simulink model "hexa_tilted_EHGO_ASMC"  (R2023a)
settings: Solver=ode1  StartTime=0.0  StopTime=tf  FixedStep=0.01  RelTol=1e-3
model workspace (MAT data in the model file):
  hover_2m = [0  0  0  0  0  0; 0  0  0  0  0  0; 2  2  2  2  2  2; 0  0  0  0  0  0; 0  0  0  0  0  0; 0  0  0  0  0  0]
  tf = Simulink.Parameter
  tf.Value = 60
  tf.DataType = 'auto'
  tf.Complexity = 'real'
  tf.Dimensions = [1 1]
  tray0 = [0  0  0  0  0  0; 0  0  0  0  0  0; 0  5  5  5  5  0; 0  0  0  0  0  0; 0  0  0  0  0  0; 0  0  0  0  0  0]
  tray1 = [0  0  0  0  0  0; 0  0  0  0  0  0; 0  5  2.5  5  2.5  0; 0  0  0  0  0  0; 0  0  0  0  0  0; 0  0  0  0  0  0]
  tray2 = [0  2  2  -2  -2  0; 0  0  -2  -2  2  0; 0  5  2.5  5  2.5  0; 0  0  0  0  0  0; 0  0  0  0  0  0; 0  0  0  0  0  0]
  tray3 = [0  2  2  -2  -2  0; 0  0  -2  -2  2  0; 0  5  2.5  5  2.5  0; 0  0  0  0  0  0; 0  0  0  0  0  0; 0  0  0.785  1.57  0.785  0]
  tray4 = [0  2  2  -2  -2  0; 0  0  -2  -2  2  0; 0  5  2.5  5  2.5  0; 0  0.15  0.15  0.15  0.15  0; 0  0  0  0  0  0; 0  0  0.785  1.57  0.785  0]
  tray5 = [0  0  0  0  0  0; 0  0  0  0  0  0; 0  5  2.5  5  2.5  0; 0  0.15  0.15  0  0  0; 0  0  0.15  0.15  0  0; 0  0  0  0  0  0]
  tray_yaw = [0  0  0  0  0  0; 0  0  0  0  0  0; 0  5  2.5  5  2.5  0; 0  0  0  0  0  0; 0  0  0  0  0  0; 0  0  0.785  1.57  0.785  0]
undefined symbols (not defined in the file or in its folder): F, Light, MIL
libraries: matrix_library x1, aerolibutil x1, simulink x1, robotcorelib x1, sharedtransform x1, aerolibwind2 x1, SignalEditorBlockLib x1
settings Model: Creator=adan  LastModifiedBy=Adan Daniel
settings OptimizationCC: ReuseModelBlockBuffer=off

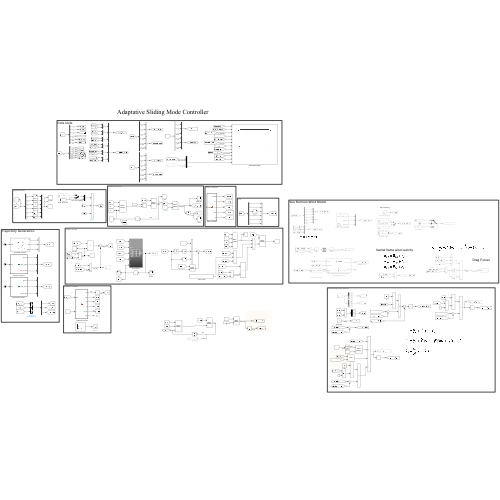
[thumbnail: Simulink's stored preview of the top-level diagram]
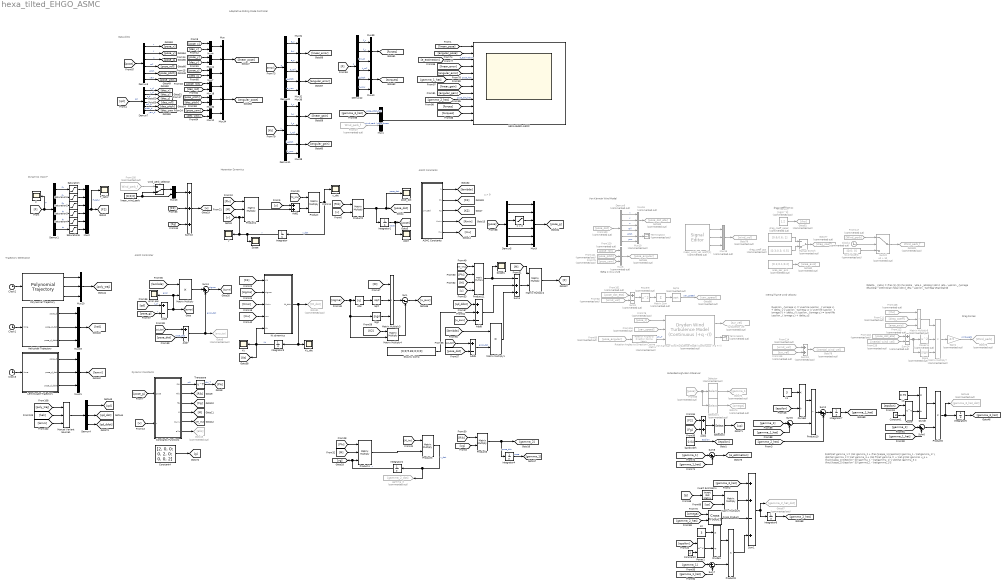
== system hexa_tilted_EHGO_ASMC ==
  note: $\dot\hat \gamma_1 = \hat \gamma_2 + \frac{\kappa_1}{\epsilon}(\gamma_1 - \hat\gamma_1) \\ \dot\hat \gamma_2 = \hat \gamma_3 + \hat f(\hat \gamma, t) + \hat g(\hat \gamma) u_p + \frac{\kappa_2}{\epsilon^2}(\gamma_1 - \hat\gamma_1) \\ \dot\hat \gamma_3 = \frac{\kappa_3}{\epsilon^3}(\gamma_1 - \hat\gamma_1)$
  note: z > 0
  note: Adaptative Sliding Mode Controller
  note: ASMC Constants
  note: ASMC Controller
  note: Dynamic Constants
  note: Hexarotor Dynamics
  note: Dynamics Input F
  note: Data plots
  note: Trajectory Generation
  note: drag coeff from []
  note: $\upsilon _{\omega x} = \overline \upsilon _{ \omega x} + \delta_u \\ \upsilon _{\omega y} = \overline \upsilon _{ \omega y} + \delta_u \\ \upsilon _{\omega z} = \overline \upsilon _{ \omega z} + \delta_u$
  note: $\eta = \{x,y,z\}$
  note: Inertial frame wind velocity
  note: $\Delta _ {\eta} = \frac{1}{2}\rho \alpha _ \eta A _\eta\big (\dot d_\eta - \upsilon _{\omega \eta}\big)^2\text{sign }\big (\dot d_\eta - \upsilon _{\omega \eta}\big)$$
  note: Von Kármán Wind Model
  note: Drag Forces
  note: Extended High-Gain Observer
  ASMC Constants : MATLAB Function  TreatAsAtomicUnit=on
  Abs : Abs  SaturateOnIntegerOverflow=off
  Add1 : Sum
  Add2 : Sum
  Add6 : Sum  Inputs=+-
  Add7 : Sum  Inputs=+-
  Add8 : Sum  Inputs=++-
  Add9 : Sum  Inputs=+-
  Clock1 : Clock
  Clock2 : Clock
  Clock3 : Clock
  Clock4 : Clock  Commented=on
  Constant1 : Constant  Value=3
  Constant2 : Constant  Value=2
  Constant4 : Constant  Value=[2, 0, 0; 0, 2, 0; 0, 0, 2]
  Constants Functions : MATLAB Function  TreatAsAtomicUnit=on
  Cross Product : matrix_library/Cross Product
  Demux{1,3,5,7..8,11..12} (7 alike) : Demux  Outputs=6
  Demux4 : Demux  Outputs=3
  Demux6 : Demux  Commented=on  Outputs=6
  Divide : Product  Inputs=*/
  Divide1 : Product  Inputs=*/
  Divide2 : Product  Inputs=*/
  F : Scope
  F_satur : Scope
  From100 : From  Commented=on  GotoTag=pose_dot
  From101 : From  Commented=on  GotoTag=pose_dot_eta
  From104 : From  Commented=on  GotoTag=uav_speed
  From105 : From  Commented=on  GotoTag=Wind_perb_f  TagVisibility=global
  From106 : From  Commented=on  GotoTag=rho
  From111 : From  Commented=on  GotoTag=drag_coeff
  From112 : From  Commented=on  GotoTag=area_axis
  From114 : From  Commented=on  GotoTag=wind_vel
  From115 : From  Commented=on  GotoTag=tur_vel
  From117 : From  Commented=on  GotoTag=Wind_perb
  From118 : From  Commented=on  GotoTag=pose_dot_eta
  From120 : From  Commented=on  GotoTag=pose_roll
  From121 : From  Commented=on  GotoTag=pose_pitch
  From126 : From  Commented=on  GotoTag=inertial_wind_vel
  From27 : From  Commented=on  GotoTag=Wind_perb_f  TagVisibility=global
  From65 : From  Commented=on  GotoTag=pose
  From75 : From  Commented=on  GotoTag=pose_yaw
  From76 : From  Commented=on  GotoTag=pose_z
  From82 : From  Commented=on  GotoTag=wind_vel
  From83 : From  Commented=on  GotoTag=pose_angular
  Gain1 : Gain  Commented=on  Gain=-0.5
  Goto15 : Goto  Commented=on  GotoTag=allo
  Goto31 : Goto  Commented=on  GotoTag=Kt_dot
  Goto39 : Goto  Commented=on  GotoTag=Wind_perb_f  TagVisibility=global
  Goto45 : Goto  Commented=on  GotoTag=gamma_3_hat_dot
  Goto6 : Goto  Commented=on  GotoTag=error_dot
  Goto67 : Goto  Commented=on  GotoTag=gamma_2_hat_dot
  Goto70 : Goto  Commented=on  GotoTag=gamma_1
  Goto74 : Goto  Commented=on  GotoTag=omega
  Goto76 : Goto  Commented=on  GotoTag=Wind_perb
  Goto77 : Goto  Commented=on  GotoTag=drag_coeff
  Goto78 : Goto  Commented=on  GotoTag=inertial_wind_vel
  Goto79 : Goto  Commented=on  GotoTag=wind_vel
  Goto80 : Goto  Commented=on  GotoTag=uav_speed
  Goto81 : Goto  Commented=on  GotoTag=rho
  Goto82 : Goto  Commented=on  GotoTag=area_axis
  Goto83 : Goto  Commented=on  GotoTag=pose_dot_eta
  Goto84 : Goto  Commented=on  GotoTag=pose_angular
  Gravity Comp : Constant  Value=[0;0;9.81;0;0;0]
  HEXA EHGO-ASMC : Scope  NumInputPorts=12
  Helicoidal Trajectory : MATLAB Function  TreatAsAtomicUnit=on
  Integrator{,1..4} (5 alike) : Integrator  InitialCondition=[0; 0; 0; 0; 0; 0]
  Integrator5 : Integrator  InitialCondition=[0; 0; 0]
  Integrator6 : Integrator  InitialCondition=[0; 0; 0]
  Integrator7 : Integrator  InitialCondition=[0; 0; 0]
  Invert 3x3 Matrix : aerolibutil/Invert  3x3 Matrix
  Kt : Scope
  Kt dynamics : Subsystem
  Kt_dot : Scope
  Lemniscate Trajectory : MATLAB Function  TreatAsAtomicUnit=on
  Manual Variant Source1 : simulink/Signal Routing/Manual Variant Source  NumChoices=3  LabelModeActiveChoice=V_2
  Manual Switch : ManualSwitch  Commented=on  CurrentSetting=0
  Matrix Sum : Sum  Commented=on  Inputs=+
  Matrix Multiply : Product
  Matrix Multiply1 : Product
  Matrix Multiply2 : Product  Multiplication=Matrix(*)
  Matrix Multiply3 : Product  Inputs=3
  Matrix Multiply4 : Product  Multiplication=Matrix(*)
  Matrix Multiply5 : Product  Multiplication=Matrix(*)
  Matrix Multiply6 : Product  Commented=on  Inputs=3
  Matrix Multiply7 : Product  Commented=on  Inputs=3
  Mux{,19..21,31..32,34,36,38..40} (11 alike) : Mux  Inputs=3
  Mux{1,4,7,11..13,18,30} (8 alike) : Mux  Inputs=2
  Mux{5,10,15..16} (4 alike) : Mux  Commented=on  Inputs=3
  Mux2 : Mux  Inputs=6
  Mux9 : Mux  Inputs=6
  Polynomial Trajectory : robotcorelib/Polynomial Trajectory  WaypointSource=Internal  Waypoints=tray1  TimePoints=[ 0, 12, 24, 36, 48, tf ]  TimeInterval=[ 1, 4 ]  Method=Cubic Polynomial  ParameterSource=Internal  VelocityBoundaryCondition=zeros( 6, 6 )  AccelerationBoundaryCondition=zeros( 2, 5 )  SimulateUsing=Interpreted execution
  Power : Math  Operator=pow
  Power1 : Math  Operator=pow
  Power11 : Math  Commented=on  Operator=square
  Power9 : Math  Commented=on  Operator=square
  Product{,2..3,5} (4 alike) : Product  Multiplication=Matrix(*)
  Product1 : Product  Inputs=3  Multiplication=Matrix(*)
  Product10 : Product
  Product11 : Product  Inputs=4  Multiplication=Matrix(*)
  Product4 : Product  Inputs=3  Multiplication=Matrix(*)
  Product6 : Product
  Product8 : Product
  Rotation Angles to Direction Cosine Matrix : sharedtransform/Rotation Angles to Direction Cosine Matrix  Commented=on  rotationOrder=ZYX  aMode=aMode
  Saturation : Saturate  UpperLimit=6  LowerLimit=-6
  Saturation1 : Saturate  UpperLimit=6  LowerLimit=-6
  Saturation2 : Saturate  UpperLimit=5.8*6  LowerLimit=0
  Saturation3 : Saturate
  Saturation4 : Saturate
  Saturation5 : Saturate
  Scope : Scope
  Scope1 : Scope
  Selector : Selector  Commented=on  InputPortWidth=6  IndexOptions=Index vector (dialog)  Indices=[1:3]  OutputSizes=1
  Selector1 : Selector  Commented=on  InputPortWidth=6  IndexOptions=Index vector (dialog)  Indices=[4:6]  OutputSizes=1
  Selector2 : Selector  InputPortWidth=6  IndexOptions=Index vector (dialog)  Indices=[1:3]  OutputSizes=1
  Sign : Signum
  Sign4 : Signum  Commented=on
  Sqrt : Sqrt
  Sqrt4 : Sqrt  Commented=on
  Sum : Sum  Inputs=|--
  Sum1 : Sum  Inputs=++-+
  Sum10 : Sum  Inputs=+++
  Sum13 : Sum  Commented=on
  Sum14 : Sum  Commented=on  Inputs=+-
  Sum2 : Sum  Inputs=|++
  Sum3 : Sum  Inputs=|++
  Sum4 : Sum  Inputs=-++
  Sum{5..8} (4 alike) : Sum  Inputs=|+-
  Sum9 : Sum  Commented=on  Inputs=+-
  Switch : Switch  Commented=on  Criteria=u2 > Threshold  Threshold=10  SaturateOnIntegerOverflow=off  InputSameDT=off
  Terminator1 : Terminator  Commented=on
  Terminator2 : Terminator  Commented=on
  Transpose : Math  Operator=transpose
  Von Karman Wind Turbulence Model (Continuous (+q +r)) : aerolibwind2/Dryden Wind Turbulence Model  (Continuous (+q -r))  Commented=on  units=Metric (MKS)  spec=MIL-F-8785C  model=Continuous Von Karman (+q -r)  W20=15  Wdeg=0  TurbProb=10^-2 - Light  L_high=762  Wingspan=10  ts=0.1  Seed=[23341 23342 23343 23344]  T_on=on
      settings: LibrarySourceBlock=|
      | aerolibwind2/Von Karman Wind Turbulence Model
      | (Continuous (+q +r))
  air density [kg/m^3] : Constant  Commented=on  Value=1.2
  area_per_axis : Constant  Commented=on  Value=[0.1;0.1;0.2]
  bandwidth : Constant  Value=0.04
  drag_coeff_gus : Constant  Commented=on  Value=[0.3;0.3; 0.5]
  drag_coeff_paper : Constant  Commented=on  Value=[0.6;0.6; 1]
  error pos : Scope
  gamma_3 : Goto  Commented=on  GotoTag=gamma_2_dot
  k1 : Constant  Value=3
  k2 : Constant  Value=3
  k3 : Constant  Value=0.75
  linear_wind_perb : Constant  Value=[0;0;0]
  mean_wind_vel_ansft[1] : SignalEditorBlockLib/Signal Editor  Commented=on  FileName=C:\Users\Adan Daniel\Documents\IMT\8Semestre_tec\Diseño e implementación de sistemas mecatronicos\mean_wind_vel_ansft.mat  ActiveScenario=Velocidades_medias_del_viento  ActiveSignal=wean_wind_vel_x  IsBus=off  OutputBusObjectStr=Bus: BusObject  SampleTime=0  Interpolate=off  ZeroCross=off  OutputAfterFinalValue=Setting to zero  Unit=inherit  PreserveSignalName=on  ApplySigPropsToAllScenarios=on
  no wind perb : Constant  Commented=on  Value=[0;0; 0]
  pose : Scope
  pose_dot : Scope
  turbulence_vel : Goto  Commented=on  GotoTag=tur_vel
  v : Scope
  v_dot : Scope
  wind_perb_selector : ManualSwitch  CurrentSetting=0
  z > 0 : Saturate  UpperLimit=100  LowerLimit=0
  wires:
  Saturation/1 -> Mux2/1
  Saturation1/1 -> Mux2/2
  Saturation4/1 -> Mux2/5
  Saturation3/1 -> Mux2/4
  Demux1/6 -> Saturation5/1  "tz"
  Demux1/3 -> Saturation2/1  "Fz"
  [F] -> F/1, Demux1/1  "F"
  Saturation5/1 -> Mux2/6
  Demux1/2 -> Saturation1/1  "Fy"
  Demux1/1 -> Saturation/1  "Fx"
  Demux1/5 -> Saturation4/1  "ty"
  Demux1/4 -> Saturation3/1  "tx"
  Saturation2/1 -> Mux2/3
  Mux2/1 -> [F2], F_satur/1  "F_satur"
  [M] -> Product1/2
  [v] -> Product2/2
  [M_inv] -> Product/1
  Add2/1 -> Product/2
  Product/1 -> v_dot/1, Integrator/1  "v_dot"
  [Rib] -> Product2/1
  Product2/1 -> Integrator1/1, pose_dot/1, [pose_dot]  "pose_dot"
  [Phi] -> Product1/1
  Product1/1 -> Add2/2
  Integrator1/1 -> pose/1, [pose]  "pose"
  Integrator/1 -> Scope/1, v/1, [v], Product1/3  "v"
  [pose_g] -> Constants Functions/1(pose)
  [v] -> Constants Functions/2(v)
  Constants Functions/6(allo) -> Goto15/1
  Constants Functions/3(Fg) -> [Fg]
  Constants Functions/4(M) -> [M]
  Constants Functions/1(Phi) -> Transpose/1  "phi"
  Constants Functions/2(Rib) -> [Rib]
  Transpose/1 -> [Phi]  "phi_T"
  Constants Functions/5(M_inv) -> [M_inv]
  [K1] -> Kt dynamics/1(K1)
  [sigma] -> Kt dynamics/2(sigma)
  [qd] -> Add6/1  "x_d"
  [Kt] -> Matrix Multiply3/1
  [mu] -> Kt dynamics/4(mu)
  Sum3/1 -> [sigma]  "sigma"
  [u_aux] -> Add8/3
  [qd_dot] -> Add9/1
  Add6/1 -> [error], Matrix Multiply/2, error pos/1  "error"
  [lambda] -> Matrix Multiply1/1
  [v] -> Product11/4  "v"
  [M] -> Matrix Multiply2/1
  Matrix Multiply4/1 -> Sum/2
  [pose_dot] -> Add9/2
  Matrix Multiply/1 -> Sum3/1
  [qd_ddot] -> Add8/1
  Add7/1 -> Goto6/1, Sum3/2  "error_dot"
  Matrix Multiply2/1 -> [F]
  [lambda] -> Matrix Multiply/1
  Sum4/1 -> Matrix Multiply2/2
  Product11/1 -> Scope1/1, Sum4/1
  [M] -> Product11/3
  Integrator3/1 -> [Kt], Kt/1, Kt dynamics/5(Kt)  "Kt"
  [pose_dot] -> Add7/2  "pose_dot"
  [K2] -> Matrix Multiply4/1
  Add9/1 -> Matrix Multiply1/2  "error_dot"
  Sign/1 -> Matrix Multiply3/3
  Abs/1 -> Sqrt/1
  [pose_g] -> Add6/2  "x"
  [M_inv] -> Product11/1
  [Kmin] -> Kt dynamics/3(Kmin)
  Add8/1 -> Sum4/2
  Matrix Multiply1/1 -> Sum4/3
  [sigma] -> Matrix Multiply4/2, Sign/1, Abs/1
  Kt dynamics/1(Kt_dot) -> Integrator3/1, Kt_dot/1, Goto31/1
  [Phi] -> Product11/2
  [qd_dot] -> Add7/1
  Matrix Multiply3/1 -> Sum/1
  Sum/1 -> [u_aux]
  ASMC Constants/4(Kmin) -> [Kmin]
  ASMC Constants/3(K2) -> [K2]
  ASMC Constants/5(mu) -> [mu]
  ASMC Constants/2(K1) -> [K1]
  ASMC Constants/1(lambda) -> [lambda]
  Sqrt/1 -> Matrix Multiply3/2
  Demux5/5 -> Mux9/5
  Demux5/6 -> Mux9/6
  Mux9/1 -> [pose_g]
  Demux5/1 -> Mux9/1
  Demux5/3 -> z > 0/1
  Demux5/2 -> Mux9/2
  Demux5/4 -> Mux9/4
  [pose] -> Demux5/1
  z > 0/1 -> Mux9/3
  Gravity Comp/1 -> Add8/2
  k3/1 -> Divide/1
  Power/1 -> Divide/2
  Constant1/1 -> Power/2
  Divide/1 -> Product6/1
  Product6/1 -> Integrator5/1, Goto45/1
  Integrator5/1 -> [gamma_3_hat]
  [des_roll] -> Mux18/2
  Mux11/1 -> Mux/2
  [des_yaw] -> Mux12/2
  [pose_pitch] -> Mux30/1
  [des_z] -> Mux7/2
  Mux4/1 -> Mux/1
  [des_pitch] -> Mux30/2
  Mux7/1 -> Mux/3
  [qd] -> Demux7/1  "qd"
  Demux3/5 -> [pose_pitch]  "pitch"
  Demux3/2 -> [pose_y]  "y"
  Demux8/4 -> Mux32/1  "e_roll"
  Demux8/2 -> Mux31/2  "e_y"
  Demux8/1 -> Mux31/1  "e_x"
  [pose_x] -> Mux4/1
  Demux3/4 -> [pose_roll]  "roll"
  Mux31/1 -> [linear_error]
  Demux7/3 -> [des_z]  "z_d"
  Mux34/1 -> [angular_pose]
  [des_y] -> Mux11/2
  Mux12/1 -> Mux34/3
  Demux3/3 -> [pose_z]  "z"
  [error] -> Demux8/1  "e"
  Demux8/5 -> Mux32/2  "e_pitch"
  [pose_yaw] -> Mux12/1
  [pose_y] -> Mux11/1
  Demux11/3 -> Mux36/3  "k_z"
  Mux30/1 -> Mux34/2
  [linear_gain] -> HEXA EHGO-ASMC/7
  Mux32/1 -> [angular_error]
  Mux38/1 -> [angular_gain]
  [forces] -> HEXA EHGO-ASMC/10
  [e_estimation] -> HEXA EHGO-ASMC/3  "e_estimation"
  Demux7/2 -> [des_y]  "y_d"
  Demux7/1 -> [des_x]  "x_d"
  [gamma_1_hat] -> HEXA EHGO-ASMC/6  "pose_hat"
  Demux12/3 -> Mux39/3  "thrust"
  [torques] -> HEXA EHGO-ASMC/11
  Demux11/4 -> Mux38/1  "k_roll"
  Demux11/5 -> Mux38/2  "k_pitch"
  [angular_pose] -> HEXA EHGO-ASMC/2
  Demux12/4 -> Mux40/1  "t_roll"
  Mux/1 -> [linear_pose]
  [pose_roll] -> Mux18/1
  Demux11/1 -> Mux36/1  "k_x"
  Demux12/5 -> Mux40/2  "t_pitch"
  [angular_error] -> HEXA EHGO-ASMC/5
  Mux18/1 -> Mux34/1
  Demux8/6 -> Mux32/3  "e_yaw"
  [angular_gain] -> HEXA EHGO-ASMC/8
  Demux7/4 -> [des_roll]  "roll_d"
  [linear_pose] -> HEXA EHGO-ASMC/1
  Mux39/1 -> [forces]
  [linear_error] -> HEXA EHGO-ASMC/4
  Demux12/1 -> Mux39/1  "f_x"
  [pose_z] -> Mux7/1
  [gamma_2_hat] -> HEXA EHGO-ASMC/9  "pose_dot_hat"
  Demux3/1 -> [pose_x]  "x"
  [Kt] -> Demux11/1  "k"
  Demux7/5 -> [des_pitch]  "pitch_d"
  [gamma_3_hat] -> Mux1/1  "pose_ddot_hat"
  Demux8/3 -> Mux31/3  "e_z"
  Mux40/1 -> [torques]
  Demux11/2 -> Mux36/2  "k_y"
  Demux7/6 -> [des_yaw]  "yaw_d"
  Demux11/6 -> Mux38/3  "k_yaw"
  Demux12/6 -> Mux40/3  "t_yaw"
  Demux12/2 -> Mux39/2  "f_y"
  [des_x] -> Mux4/2
  Mux36/1 -> [linear_gain]
  [F] -> Demux12/1  "f"
  Demux3/6 -> [pose_yaw]  "yaw"
  [pose] -> Demux3/1
  [gamma_3_hat] -> Sum1/1
  Constant2/1 -> Power1/2
  k2/1 -> Divide1/1
  Power1/1 -> Divide1/2
  [epsilon] -> Power1/1
  Divide1/1 -> Product8/1
  Product8/1 -> Sum1/4
  Sum1/1 -> Integrator6/1, Goto67/1
  Integrator6/1 -> [gamma_2_hat]
  k1/1 -> Divide2/1
  Divide2/1 -> Product10/1
  [epsilon] -> Divide2/2
  Product10/1 -> Sum2/1
  [gamma_2_hat] -> Sum2/2
  Sum2/1 -> Integrator7/1
  Integrator7/1 -> [gamma_1_hat]
  [gamma_1_hat] -> Sum5/2
  Sum5/1 -> Product10/2
  [gamma_1] -> Sum5/1
  Sum6/1 -> Product6/2
  [gamma_1_hat] -> Sum6/2
  [gamma_1] -> Sum6/1
  Sum7/1 -> Product8/2
  [gamma_1_hat] -> Sum7/2
  [gamma_1] -> Sum7/1
  [F2] -> Add1/1
  Add1/1 -> Selector2/1
  [Fg] -> Add1/2
  Polynomial Trajectory/3 -> Mux20/3
  Helicoidal Trajectory/1(pose_d) -> Mux19/1
  Polynomial Trajectory/1 -> Mux20/1
  Helicoidal Trajectory/2(pose_d_dot) -> Mux19/2
  Mux19/1 -> [heli]
  Demux4/2 -> [qd_dot]
  Mux20/1 -> [poly_traj]
  Lemniscate Trajectory/3(pose_d_ddot) -> Mux21/3
  Clock1/1 -> Helicoidal Trajectory/1(time)
  Clock2/1 -> Polynomial Trajectory/1
  Demux4/3 -> [qd_ddot]
  Clock3/1 -> Lemniscate Trajectory/1(time)
  Helicoidal Trajectory/3(pose_d_ddot) -> Mux19/3
  [lemni] -> Manual Variant Source1/3
  [poly_traj] -> Manual Variant Source1/1
  [heli] -> Manual Variant Source1/2
  Lemniscate Trajectory/1(pose_d) -> Mux21/1
  Lemniscate Trajectory/2(pose_d_dot) -> Mux21/2
  Polynomial Trajectory/2 -> Mux20/2
  Demux4/1 -> [qd]
  Mux21/1 -> [lemni]
  Manual Variant Source1/1 -> Demux4/1
  From65/1 -> Selector1/1, Selector/1
  Selector/1 -> Goto70/1
  [up] -> Matrix Multiply5/2
  Constant4/1 -> [g]
  [g] -> Invert 3x3 Matrix/1
  Invert 3x3 Matrix/1 -> Matrix Multiply5/1
  Matrix Multiply5/1 -> Sum1/2
  Selector1/1 -> Goto74/1
  [omega] -> Cross Product/1
  [gamma_2_hat] -> Cross Product/2
  Cross Product/1 -> Sum1/3
  Selector2/1 -> [up]
  Sum8/1 -> [e_estimation]
  [gamma_1_hat] -> Sum8/2
  [gamma_1] -> Sum8/1
  Power11/1 -> Matrix Multiply7/2
  Sqrt4/1 -> Goto80/1  "uav_speed"
  Demux6/5 -> Mux10/2  "pitch"
  From115/1 -> Sum13/2
  From112/1 -> Matrix Multiply6/3
  Demux6/6 -> Mux10/3  "yaw"
  mean_wind_vel_ansft[1]/1 -> Mux15/1
  From121/1 -> Mux5/2
  Demux6/4 -> Mux10/1  "roll"
  Power9/1 -> Matrix Sum/1
  From82/1 -> Sum9/2
  From126/1 -> Sum14/2
  Von Karman Wind Turbulence Model (Continuous (+q +r))/1 -> turbulence_vel/1
  Matrix Sum/1 -> Sqrt4/1
  Mux15/1 -> Goto79/1
  Matrix Multiply7/1 -> Gain1/1
  From118/1 -> Sum14/1
  Rotation Angles to Direction Cosine Matrix/1 -> Von Karman Wind Turbulence Model (Continuous (+q +r))/3  "phi_T"
  drag_coeff_paper/1 -> Manual Switch/1
  Mux16/1 -> Goto83/1
  area_per_axis/1 -> Goto82/1
  Gain1/1 -> Goto76/1  "wind_perb"
  From120/1 -> Mux5/1
  Manual Switch/1 -> Goto77/1
  From101/1 -> Sum9/1
  From75/1 -> Mux5/3
  mean_wind_vel_ansft[1]/2 -> Mux15/2
  Demux6/3 -> Mux16/3  "z"
  Mux5/1 -> Goto84/1
  Sum13/1 -> Goto78/1
  From76/1 -> Von Karman Wind Turbulence Model (Continuous (+q +r))/1
  From114/1 -> Sum13/1
  From117/1 -> Switch/1
  Matrix Multiply6/1 -> Matrix Multiply7/1
  Von Karman Wind Turbulence Model (Continuous (+q +r))/2 -> Terminator1/1
  From83/1 -> Rotation Angles to Direction Cosine Matrix/1
  air density [kg/m^3]/1 -> Goto81/1
  From104/1 -> Von Karman Wind Turbulence Model (Continuous (+q +r))/2
  Mux10/1 -> Terminator2/1
  Demux6/1 -> Mux16/1  "x"
  Sum14/1 -> Sign4/1, Power11/1
  no wind perb/1 -> Switch/3
  From106/1 -> Matrix Multiply6/1
  From100/1 -> Demux6/1
  From111/1 -> Matrix Multiply6/2
  Switch/1 -> Goto39/1
  drag_coeff_gus/1 -> Manual Switch/2
  mean_wind_vel_ansft[1]/3 -> Mux15/3
  Clock4/1 -> Switch/2
  Sign4/1 -> Matrix Multiply7/3
  Sum9/1 -> Power9/1
  Demux6/2 -> Mux16/2  "y"
  bandwidth/1 -> [epsilon]  "epsilon"
  [epsilon] -> Power/1
  From27/1 -> Mux1/2  "wind perb | drag forces"
  Mux1/1 -> HEXA EHGO-ASMC/12
  [vg] -> Product5/2
  Product3/1 -> gamma_3/1, Integrator2/1  "v_dot"
  [M] -> Product4/2
  [M_inv] -> Product3/1
  [Phi] -> Product4/1
  Product4/1 -> Product3/2
  Product5/1 -> Integrator4/1, [gamma_2]  "pose_dot"
  Integrator4/1 -> [gamma_1]  "pose"
  Integrator2/1 -> [vg], Product4/3  "v"
  [Rib] -> Product5/1
  linear_wind_perb/1 -> Mux13/2, wind_perb_selector/2
  From105/1 -> wind_perb_selector/1
  wind_perb_selector/1 -> Mux13/1
  Mux13/1 -> Sum10/1
  [F2] -> Sum10/2
  [Fg] -> Sum10/3
  Sum10/1 -> [u]
  [u] -> Add2/1

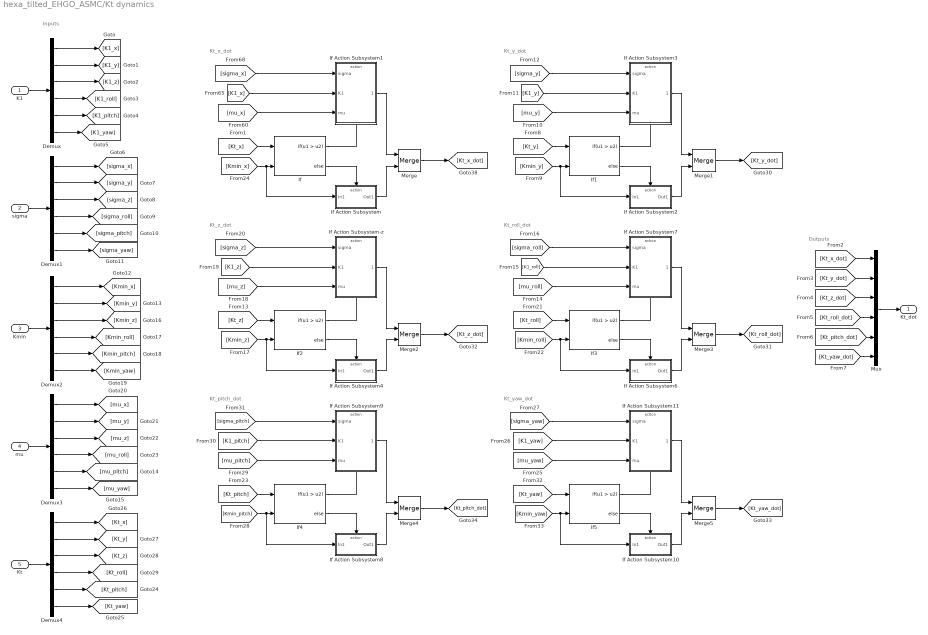
== system hexa_tilted_EHGO_ASMC/Kt dynamics ==
  note: Outputs
  note: Inputs
  note: Kt_x_dot
  note: Kt_y_dot
  note: Kt_z_dot
  note: Kt_roll_dot
  note: Kt_pitch_dot
  note: Kt_yaw_dot
  K1 : Inport
  sigma : Inport  Port=2
  Kmin : Inport  Port=3
  mu : Inport  Port=4
  Kt : Inport  Port=5
  Demux{,1..4} (5 alike) : Demux  Outputs=6
  If{,1..5} (6 alike) : If  NumInputs=2  IfExpression=u1 > u2
  If Action Subsystem : Subsystem  TreatAsAtomicUnit=on
  If Action Subsystem-z : Subsystem  TreatAsAtomicUnit=on
  If Action Subsystem1 : Subsystem  TreatAsAtomicUnit=on
  If Action Subsystem10 : Subsystem  TreatAsAtomicUnit=on
  If Action Subsystem11 : Subsystem  TreatAsAtomicUnit=on
  If Action Subsystem2 : Subsystem  TreatAsAtomicUnit=on
  If Action Subsystem3 : Subsystem  TreatAsAtomicUnit=on
  If Action Subsystem4 : Subsystem  TreatAsAtomicUnit=on
  If Action Subsystem6 : Subsystem  TreatAsAtomicUnit=on
  If Action Subsystem7 : Subsystem  TreatAsAtomicUnit=on
  If Action Subsystem8 : Subsystem  TreatAsAtomicUnit=on
  If Action Subsystem9 : Subsystem  TreatAsAtomicUnit=on
  Merge{,1..5} (6 alike) : Merge
  Mux : Mux  Inputs=6
  Kt_dot : Outport
  wires:
  [Kt_x] -> If/1
  [sigma_x] -> If Action Subsystem1/1(sigma)
  If/1 -> If Action Subsystem1/Action
  [K1_x] -> If Action Subsystem1/2(K1)
  If Action Subsystem1/1(Kt_x_dot) -> Merge/1
  If Action Subsystem/1(Out1) -> Merge/2
  If/2 -> If Action Subsystem/Action
  Merge/1 -> [Kt_x_dot]
  [Kmin_x] -> If Action Subsystem/1(In1), If/2
  [mu_x] -> If Action Subsystem1/3(mu)
  Merge1/1 -> [Kt_y_dot]
  If1/2 -> If Action Subsystem2/Action
  If Action Subsystem2/1(Out1) -> Merge1/2
  If Action Subsystem3/1(Kt_x_dot) -> Merge1/1
  [Kt_y] -> If1/1
  [K1_y] -> If Action Subsystem3/2(K1)
  [mu_y] -> If Action Subsystem3/3(mu)
  [Kmin_y] -> If Action Subsystem2/1(In1), If1/2
  [sigma_y] -> If Action Subsystem3/1(sigma)
  Merge2/1 -> [Kt_z_dot]
  If Action Subsystem-z/1(Kt_z_dot) -> Merge2/1
  [sigma_z] -> If Action Subsystem-z/1(sigma)
  [Kt_z] -> If2/1
  [mu_z] -> If Action Subsystem-z/3(mu)
  [Kmin_z] -> If Action Subsystem4/1(In1), If2/2
  If3/2 -> If Action Subsystem6/Action
  If Action Subsystem7/1(Kt_x_dot) -> Merge3/1
  Merge3/1 -> [Kt_roll_dot]
  If3/1 -> If Action Subsystem7/Action
  [Kmin_roll] -> If Action Subsystem6/1(In1), If3/2
  If2/2 -> If Action Subsystem4/Action
  [sigma_roll] -> If Action Subsystem7/1(sigma)
  If2/1 -> If Action Subsystem-z/Action
  [K1_roll] -> If Action Subsystem7/2(K1)
  If Action Subsystem6/1(Out1) -> Merge3/2
  [mu_roll] -> If Action Subsystem7/3(mu)
  If Action Subsystem4/1(Out1) -> Merge2/2
  [Kt_roll] -> If3/1
  [K1_z] -> If Action Subsystem-z/2(K1)
  Merge4/1 -> [Kt_pitch_dot]
  If Action Subsystem9/1(Kt_x_dot) -> Merge4/1
  [sigma_pitch] -> If Action Subsystem9/1(sigma)
  [Kt_pitch] -> If4/1
  [mu_pitch] -> If Action Subsystem9/3(mu)
  [Kmin_pitch] -> If Action Subsystem8/1(In1), If4/2
  If5/2 -> If Action Subsystem10/Action
  If Action Subsystem11/1(Kt_x_dot) -> Merge5/1
  Merge5/1 -> [Kt_yaw_dot]
  If5/1 -> If Action Subsystem11/Action
  [Kmin_yaw] -> If Action Subsystem10/1(In1), If5/2
  If4/2 -> If Action Subsystem8/Action
  [sigma_yaw] -> If Action Subsystem11/1(sigma)
  If4/1 -> If Action Subsystem9/Action
  [K1_yaw] -> If Action Subsystem11/2(K1)
  If Action Subsystem10/1(Out1) -> Merge5/2
  [mu_yaw] -> If Action Subsystem11/3(mu)
  If Action Subsystem8/1(Out1) -> Merge4/2
  [Kt_yaw] -> If5/1
  [K1_pitch] -> If Action Subsystem9/2(K1)
  If1/1 -> If Action Subsystem3/Action
  Demux4/6 -> [Kt_yaw]
  Demux4/1 -> [Kt_x]
  Demux1/5 -> [sigma_pitch]
  Demux1/3 -> [sigma_z]
  Demux1/1 -> [sigma_x]
  Demux1/2 -> [sigma_y]
  Kt/1 -> Demux4/1
  Demux4/4 -> [Kt_roll]
  sigma/1 -> Demux1/1
  Demux3/4 -> [mu_roll]
  Demux2/4 -> [Kmin_roll]
  Demux3/1 -> [mu_x]
  Demux2/3 -> [Kmin_z]
  Demux3/3 -> [mu_z]
  mu/1 -> Demux3/1
  Demux3/6 -> [mu_yaw]
  Demux3/5 -> [mu_pitch]
  Demux2/5 -> [Kmin_pitch]
  Demux3/2 -> [mu_y]
  Demux2/6 -> [Kmin_yaw]
  Demux2/1 -> [Kmin_x]
  Demux2/2 -> [Kmin_y]
  Demux/4 -> [K1_roll]
  Demux1/4 -> [sigma_roll]
  Demux4/5 -> [Kt_pitch]
  Demux4/2 -> [Kt_y]
  Demux4/3 -> [Kt_z]
  Demux/1 -> [K1_x]
  K1/1 -> Demux/1
  Demux/6 -> [K1_yaw]
  Demux/5 -> [K1_pitch]
  Demux1/6 -> [sigma_yaw]
  Demux/2 -> [K1_y]
  Kmin/1 -> Demux2/1
  Demux/3 -> [K1_z]
  Mux/1 -> Kt_dot/1
  [Kt_z_dot] -> Mux/3
  [Kt_yaw_dot] -> Mux/6
  [Kt_pitch_dot] -> Mux/5
  [Kt_x_dot] -> Mux/1
  [Kt_y_dot] -> Mux/2
  [Kt_roll_dot] -> Mux/4

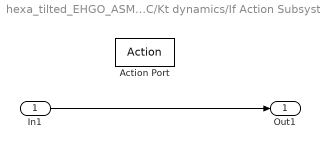
== system hexa_tilted_EHGO_ASMC/Kt dynamics/If Action Subsystem ==
  In1 : Inport
  Action Port : ActionPort  ActionPortLabel=else
  Out1 : Outport
  wires:
  In1/1 -> Out1/1

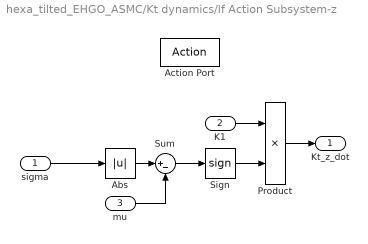
== system hexa_tilted_EHGO_ASMC/Kt dynamics/If Action Subsystem-z ==
  sigma : Inport
  K1 : Inport  Port=2
  mu : Inport  Port=3
  Action Port : ActionPort  ActionPortLabel=if(u1 > u2)
  Abs : Abs  SaturateOnIntegerOverflow=off
  Product : Product
  Sign : Signum
  Sum : Sum  Inputs=|+-
  Kt_z_dot : Outport
  wires:
  sigma/1 -> Abs/1
  Abs/1 -> Sum/1
  mu/1 -> Sum/2
  Sum/1 -> Sign/1
  Product/1 -> Kt_z_dot/1
  Sign/1 -> Product/2
  K1/1 -> Product/1

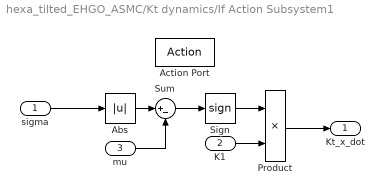
== system hexa_tilted_EHGO_ASMC/Kt dynamics/If Action Subsystem1 ==
  sigma : Inport
  K1 : Inport  Port=2
  mu : Inport  Port=3
  Action Port : ActionPort  ActionPortLabel=if(u1 > u2)
  Abs : Abs  SaturateOnIntegerOverflow=off
  Product : Product
  Sign : Signum
  Sum : Sum  Inputs=|+-
  Kt_x_dot : Outport
  wires:
  sigma/1 -> Abs/1
  Abs/1 -> Sum/1
  mu/1 -> Sum/2
  Sum/1 -> Sign/1
  Sign/1 -> Product/1
  K1/1 -> Product/2
  Product/1 -> Kt_x_dot/1

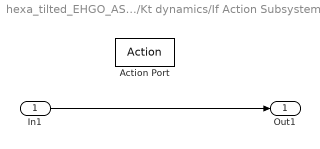
== system hexa_tilted_EHGO_ASMC/Kt dynamics/If Action Subsystem10 ==
  In1 : Inport
  Action Port : ActionPort  ActionPortLabel=else
  Out1 : Outport
  wires:
  In1/1 -> Out1/1

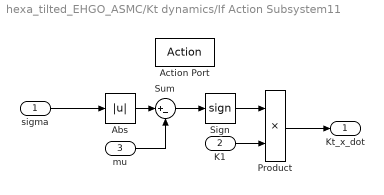
== system hexa_tilted_EHGO_ASMC/Kt dynamics/If Action Subsystem11 ==
  sigma : Inport
  K1 : Inport  Port=2
  mu : Inport  Port=3
  Action Port : ActionPort  ActionPortLabel=if(u1 > u2)
  Abs : Abs  SaturateOnIntegerOverflow=off
  Product : Product
  Sign : Signum
  Sum : Sum  Inputs=|+-
  Kt_x_dot : Outport
  wires:
  sigma/1 -> Abs/1
  Abs/1 -> Sum/1
  mu/1 -> Sum/2
  Sum/1 -> Sign/1
  Sign/1 -> Product/1
  K1/1 -> Product/2
  Product/1 -> Kt_x_dot/1

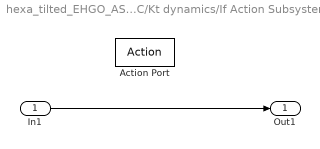
== system hexa_tilted_EHGO_ASMC/Kt dynamics/If Action Subsystem2 ==
  In1 : Inport
  Action Port : ActionPort  ActionPortLabel=else
  Out1 : Outport
  wires:
  In1/1 -> Out1/1

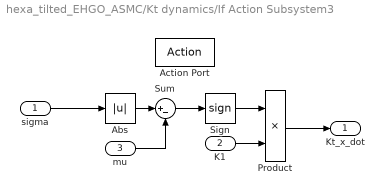
== system hexa_tilted_EHGO_ASMC/Kt dynamics/If Action Subsystem3 ==
  sigma : Inport
  K1 : Inport  Port=2
  mu : Inport  Port=3
  Action Port : ActionPort  ActionPortLabel=if(u1 > u2)
  Abs : Abs  SaturateOnIntegerOverflow=off
  Product : Product
  Sign : Signum
  Sum : Sum  Inputs=|+-
  Kt_x_dot : Outport
  wires:
  sigma/1 -> Abs/1
  Abs/1 -> Sum/1
  mu/1 -> Sum/2
  Sum/1 -> Sign/1
  Sign/1 -> Product/1
  K1/1 -> Product/2
  Product/1 -> Kt_x_dot/1

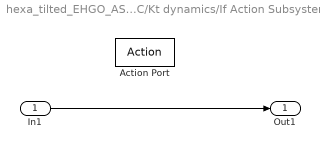
== system hexa_tilted_EHGO_ASMC/Kt dynamics/If Action Subsystem4 ==
  In1 : Inport
  Action Port : ActionPort  ActionPortLabel=else
  Out1 : Outport
  wires:
  In1/1 -> Out1/1

== system hexa_tilted_EHGO_ASMC/Kt dynamics/If Action Subsystem6 ==
  In1 : Inport
  Action Port : ActionPort  ActionPortLabel=else
  Out1 : Outport
  wires:
  In1/1 -> Out1/1

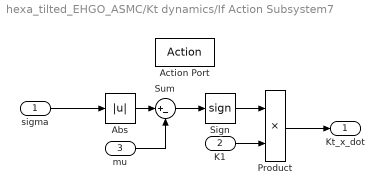
== system hexa_tilted_EHGO_ASMC/Kt dynamics/If Action Subsystem7 ==
  sigma : Inport
  K1 : Inport  Port=2
  mu : Inport  Port=3
  Action Port : ActionPort  ActionPortLabel=if(u1 > u2)
  Abs : Abs  SaturateOnIntegerOverflow=off
  Product : Product
  Sign : Signum
  Sum : Sum  Inputs=|+-
  Kt_x_dot : Outport
  wires:
  sigma/1 -> Abs/1
  Abs/1 -> Sum/1
  mu/1 -> Sum/2
  Sum/1 -> Sign/1
  Sign/1 -> Product/1
  K1/1 -> Product/2
  Product/1 -> Kt_x_dot/1

== system hexa_tilted_EHGO_ASMC/Kt dynamics/If Action Subsystem8 ==
  In1 : Inport
  Action Port : ActionPort  ActionPortLabel=else
  Out1 : Outport
  wires:
  In1/1 -> Out1/1

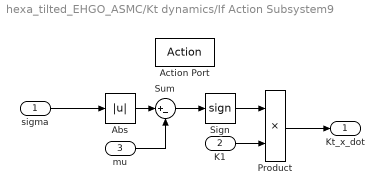
== system hexa_tilted_EHGO_ASMC/Kt dynamics/If Action Subsystem9 ==
  sigma : Inport
  K1 : Inport  Port=2
  mu : Inport  Port=3
  Action Port : ActionPort  ActionPortLabel=if(u1 > u2)
  Abs : Abs  SaturateOnIntegerOverflow=off
  Product : Product
  Sign : Signum
  Sum : Sum  Inputs=|+-
  Kt_x_dot : Outport
  wires:
  sigma/1 -> Abs/1
  Abs/1 -> Sum/1
  mu/1 -> Sum/2
  Sum/1 -> Sign/1
  Sign/1 -> Product/1
  K1/1 -> Product/2
  Product/1 -> Kt_x_dot/1

== matlab function hexa_tilted_EHGO_ASMC/Helicoidal Trajectory ==
  data: time input; pose_d output; pose_d_dot output; pose_d_ddot output
function [pose_d, pose_d_dot, pose_d_ddot]= fcn(time)

pos_z = time / 12;

% hover for 5 s | include inclination in roll

if (time < 5)
    pos_x = 0;
    pos_y = 0;
    roll = 0;
elseif (time >= 5 && time < 30)
    pos_x = 1.2 * cos (0.25 * (time - 5));
    pos_y = 1.2 * sin (0.25 * (time - 5));
    roll = 0;
else
    roll = 0.15;
    pos_x = 1.2 * cos (0.25 * (time - 5));
    pos_y = 1.2 * sin (0.25 * (time - 5));
end

% roll = 0;
yaw = time * 0;

pose_d = [pos_x;
          pos_y;
          pos_z;
          roll;
          0;
          yaw];

pos_z_dot = 1 / 12;

% hover for 5 s
if (time < 5)
    pos_x_dot = 0;
    pos_y_dot = 0;
else
    pos_x_dot = - 0.25 * 1.2 * sin(0.25 * (time - 5));
    pos_y_dot = 0.25 * 1.2 * cos(0.25 * (time - 5));
end

yaw_dot = 0;

pose_d_dot = [pos_x_dot;
              pos_y_dot;
              pos_z_dot;
              0;
              0;
              yaw_dot];

pos_z_ddot = 0;
% hover for 5 s
if (time < 5)
    pos_x_ddot = 0;
    pos_y_ddot = 0;
else
    pos_x_ddot = - 0.25 * 0.25 * 1.2 * cos(0.25 * (time - 5));
    pos_y_ddot = - 0.25 * 0.25 * 1.2 * sin(0.25 * (time - 5));
end

yaw_ddot = 0;

pose_d_ddot = [pos_x_ddot;
               pos_y_ddot;
               pos_z_ddot;
               0;
               0;
               yaw_ddot];

== matlab function hexa_tilted_EHGO_ASMC/ASMC Constants ==
  data: unused input; lambda output; K1 output; K2 output; Kmin output; mu output
function [lambda, K1, K2, Kmin, mu] = fcn(~)

% valores de lambda > 0
% entre más grande agrega estrés al sistema
lambda = [5; 5; 10; 10; 10; 10];

% valores de K > 0
%K = [7.5; 7.5; 15; 5; 5; 5];

K1  = [1.5; 2.5; 5; 0.25; 0.25; 0.1];

K2 = [0.01, 0, 0, 0, 0, 0;
     0, 0.01, 0, 0, 0, 0;
     0, 0, 0.001, 0, 0, 0;
     0, 0, 0, 10, 0, 0;
     0, 0, 0, 0, 10, 0;
     0, 0, 0, 0, 0, 5];

Kmin = [0.05; 0.05; 1; 0.1; 0.01; 0.01];

mu = [0.05; 0.05; 0.01; 0.01; 0.01; 0.1];

== matlab function hexa_tilted_EHGO_ASMC/Constants Functions ==
  data: Phi output; Rib output; Fg output; pose input; M output; M_inv output; allo output; v input
function [Phi, Rib, Fg, M, M_inv, allo] = fcn(pose, v)

%% system constants
pi = 3.141592;
m = 2.0; %5 mass 2.2 kg
l = 0.25; % length m
g = 9.81; % gravity m/s²
Jxx =  24778420.82/(1000*1000000); % kg m²
Jyy = 42217933.96/(1000*1000000); % kg m²
Jzz = 23948304.24/(1000*1000000); % kg m²
kT = 0.000006975938113;
kQ = 0.000118290418538;

%% Phi matrix calculation
uu = v(1);
vv = v(2);
ww = v(3);
pp = v(4);
qq = v(5);
rr = v(6);


Phi = [0, -rr, qq, 0, -ww, vv;
        rr, 0, -pp , ww, 0, -uu;
        -qq, pp, 0,  -vv, uu, 0;
        0, 0, 0, 0, -rr, qq; 
        0, 0, 0, rr, 0, -pp;
        0, 0, 0, -qq, pp, 0];

%% Rib matrix calculation

roll = pose(4);
pitch = pose(5);
yaw = pose(6);

Rib = [cos(yaw)*cos(pitch), -cos(roll)*sin(yaw) + cos(yaw)*sin(roll)*sin(pitch), sin(roll)*sin(yaw) + cos(roll)*cos(yaw)*sin(pitch), 0, 0, 0;
       cos(pitch)*sin(yaw), cos(roll)*cos(yaw) + sin(yaw)*sin(pitch)*sin(roll), -cos(yaw)*sin(roll) + sin(yaw)*sin(pitch)*cos(roll), 0, 0, 0;
       -sin(pitch), cos(pitch)*sin(roll), cos(pitch)*cos(roll), 0, 0, 0;
       0, 0, 0, 1, sin(roll)*tan(pitch), cos(roll)*tan(pitch);
       0, 0, 0, 0, cos(roll), -sin(roll);
       0, 0, 0, 0, sin(roll)/cos(pitch), cos(roll)/cos(pitch)];

%% Fg matrix calculation

Fg = [m*g*sin(pitch);
      -m*g*cos(pitch)*sin(roll);
      -m*g*cos(pitch)*cos(roll);
      0;
      0;
      0];

M = [m, 0, 0, 0, 0, 0;
    0, m, 0, 0, 0, 0;
    0, 0, m, 0, 0, 0;
    0, 0, 0, Jxx, 0, 0;
    0, 0, 0, 0, Jyy, 0;
    0, 0, 0, 0, 0, Jzz];

M_inv = inv(M);

alpha = [pi/6; -pi/6; -pi/2; -5*pi/6; 5*pi/6; pi/2];

varphi = pi/9;

%% tilted rotors matrix allocation

m11 = -kT*cos(alpha(1))*sin(varphi);
m21 = kT*sin(alpha(1))*sin(varphi);
m31 = kT*cos(varphi);
m41 = cos(alpha(1))*(l*kT*cos(varphi) - kQ*sin(varphi));
m51 = sin(alpha(1))*(-l*kT*cos(varphi) + kQ*sin(varphi));
m61 = l*kT*sin(varphi) + kQ*cos(varphi);

m12 = kT*cos(alpha(2))*sin(varphi);
m22 = -kT*sin(alpha(2))*sin(varphi);
m32 = m31;
m42 = cos(alpha(2))*(l*kT*cos(varphi) - kQ*sin(varphi));
m52 = sin(alpha(2))*(-l*kT*cos(varphi) + kQ*sin(varphi));
m62 = -l*kT*sin(varphi) - kQ*cos(varphi);

m13 = kT*cos(alpha(3))*sin(varphi);
m23 = kT*sin(alpha(3))*sin(varphi);
m33 = m31;
m43 = cos(alpha(3))*(l*kT*cos(varphi) + kQ*sin(varphi));
m53 = sin(alpha(3))*(-l*kT*cos(varphi) + kQ*sin(varphi));
m63 = l*kT*sin(varphi) + kQ*cos(varphi);

m14 = kT*cos(alpha(4))*sin(varphi);
m24 = -kT*sin(alpha(4))*sin(varphi);
m34 = m31;
m44 = cos(alpha(4))*(l*kT*cos(varphi) - kQ*sin(varphi));
m54 = sin(alpha(4))*(-l*kT*cos(varphi) + kQ*sin(varphi));
m64 = -l*kT*sin(varphi) - kQ*cos(varphi);

m15 = -kT*cos(alpha(5))*sin(varphi);
m25 = kT*sin(alpha(5))*sin(varphi);
m35 = m31;
m45 = cos(alpha(5))*(l*kT*cos(varphi) - kQ*sin(varphi));
m55 = sin(alpha(5))*(-l*kT*cos(varphi) + kQ*sin(varphi));
m65 = l*kT*sin(varphi) + kQ*cos(varphi);

m16 = kT*cos(alpha(6))*sin(varphi);
m26 = -kT*sin(alpha(6))*sin(varphi);
m36 = m31;
m46 = cos(alpha(6))*(l*kT*cos(varphi) + kQ*sin(varphi));
m56 = sin(alpha(6))*(-l*kT*cos(varphi) + kQ*sin(varphi));
m66 = -l*kT*sin(varphi) - kQ*cos(varphi);

allo = [m11, m12, m13, m14, m15, m16;
        m21, m22, m23, m24, m25, m26;
        m31, m32, m33, m34, m35, m36;
        m41, m42, m43, m44, m45, m46;
        m51, m52, m53, m54, m55, m56;
        m61, m62, m63, m64, m65, m66];

allo = inv(allo);

== matlab function hexa_tilted_EHGO_ASMC/Lemniscate Trajectory ==
  data: time input; pose_d output; pose_d_dot output; pose_d_ddot output
function [pose_d, pose_d_dot, pose_d_ddot]= fcn(time)

%% Positions

arg = time / 4;

pos_x = cos(arg) ./ (1 + sin(arg) .* sin(arg));
pos_y = cos(arg) .* sin(arg) ./ (1 + sin(arg) .* sin(arg));
pos_z = time / 12;

yaw = time * 0;

pose_d = [pos_x;
          pos_y;
          pos_z;
          0;
          0;
          yaw];

%% Velocities

pos_z_dot = 1 / 12;
pos_x_dot = 0;
pos_y_dot = 0;
yaw_dot = 0;

pose_d_dot = [pos_x_dot;
              pos_y_dot;
              pos_z_dot;
              0;
              0;
              yaw_dot];

%% Accelerations

pos_z_ddot = 0;
pos_x_ddot = 0;
pos_y_ddot = 0;
yaw_ddot = 0;

pose_d_ddot = [pos_x_ddot;
               pos_y_ddot;
               pos_z_ddot;
               0;
               0;
               yaw_ddot];
